simulink model "secondmodel"  (R2022b)
settings: Solver=VariableStepAuto  StartTime=0.0  StopTime=200  RelTol=1e-3
undefined symbols (not defined in the file): kr, Tp
settings Model: Creator=Chyba Ja  LastModifiedBy=janro
settings DebuggingCC: UnconnectedInputMsg=warning  UnconnectedOutputMsg=warning  UnconnectedLineMsg=warning
settings ModelReferenceCC: EnableRefExpFcnMdlSchedulingChecks=on
settings RTWCC: DLArmComputeVersion=19.05

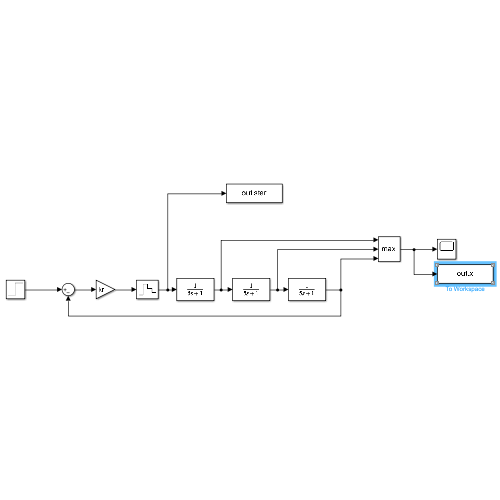
[thumbnail: Simulink's stored preview of the top-level diagram]
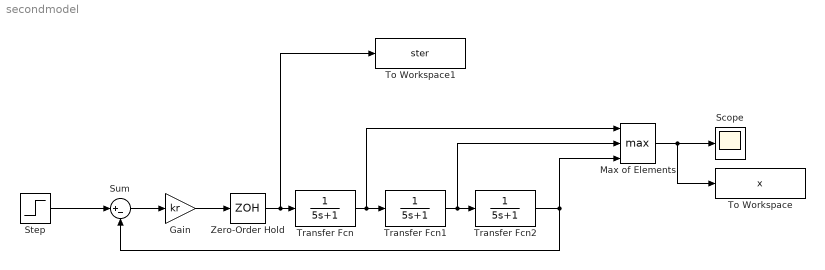
== system secondmodel ==
  Gain : Gain  Gain=kr
  Max of Elements : MinMax  Function=max  Inputs=3
  Scope : Scope
  Step : Step  SampleTime=0
  Sum : Sum  Inputs=|+-
  To Workspace : ToWorkspace  VariableName=x  SaveFormat=Timeseries  SampleTime=-1
  To Workspace1 : ToWorkspace  VariableName=ster  SaveFormat=Timeseries  SampleTime=-1
  Transfer Fcn : TransferFcn  Denominator=[5 1]
  Transfer Fcn1 : TransferFcn  Denominator=[5 1]
  Transfer Fcn2 : TransferFcn  Denominator=[5 1]
  Zero-Order Hold : ZeroOrderHold  SampleTime=Tp
  wires:
  Sum/1 -> Gain/1
  Step/1 -> Sum/1
  Gain/1 -> Zero-Order Hold/1
  Zero-Order Hold/1 -> To Workspace1/1, Transfer Fcn/1
  Transfer Fcn1/1 -> Max of Elements/2, Transfer Fcn2/1
  Transfer Fcn/1 -> Max of Elements/1, Transfer Fcn1/1
  Max of Elements/1 -> To Workspace/1, Scope/1
  Transfer Fcn2/1 -> Sum/2, Max of Elements/3
